simulink model "Simulink_System2"  (R2020a)
settings: Solver=VariableStepAuto  StartTime=0.0  StopTime=50  MaxStep=0.001  RelTol=1e-3
undefined symbols (not defined in the file): a, k2, kcA2, kcSO2, kdA2, kdSO2, kiA2, kiSO2
libraries: cstblocks x4, simulink x1
settings Model: Creator=beto1  LastModifiedBy=beto1

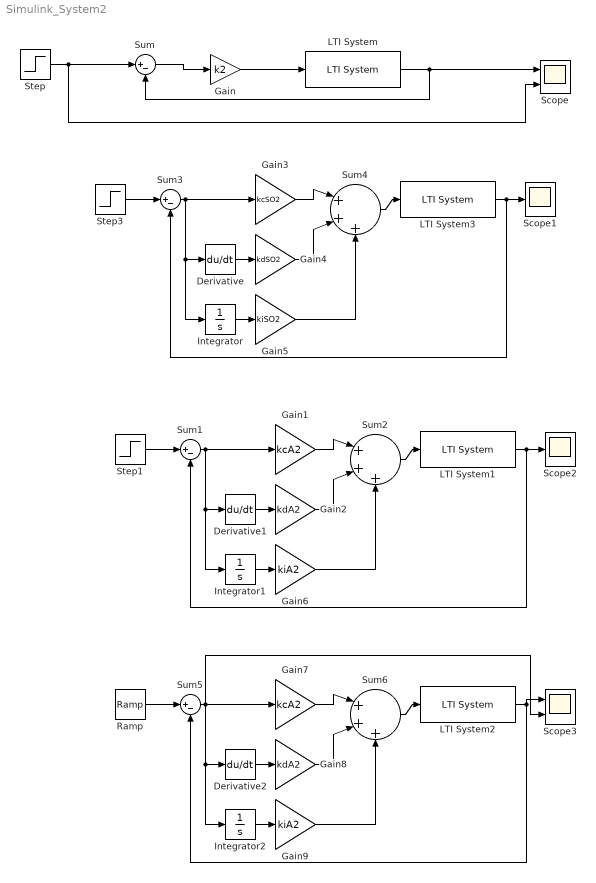
== system Simulink_System2 ==
  Derivative : Derivative
  Derivative1 : Derivative
  Derivative2 : Derivative
  Gain : Gain  Gain=k2
  Gain1 : Gain  Gain=kcA2
  Gain2 : Gain  Gain=kdA2
  Gain3 : Gain  Gain=kcSO2
  Gain4 : Gain  Gain=kdSO2
  Gain5 : Gain  Gain=kiSO2
  Gain6 : Gain  Gain=kiA2
  Gain7 : Gain  Gain=kcA2
  Gain8 : Gain  Gain=kdA2
  Gain9 : Gain  Gain=kiA2
  Integrator : Integrator
  Integrator1 : Integrator
  Integrator2 : Integrator
  LTI System{,1..3} (4 alike) : cstblocks/LTI System  sys=G2  IC=[]
  Ramp : simulink/Sources/Ramp  slope=a  start=0  InitialOutput=0
  Scope : Scope  NumInputPorts=2
  Scope1 : Scope
  Scope2 : Scope
  Scope3 : Scope  NumInputPorts=2
  Step : Step  Time=0  SampleTime=0
  Step1 : Step  Time=0  After=8  SampleTime=0
  Step3 : Step  Time=0  After=8  SampleTime=0
  Sum{,1,3,5} (4 alike) : Sum  Inputs=|+-
  Sum2 : Sum  Inputs=|+++
  Sum4 : Sum  Inputs=|+++
  Sum6 : Sum  Inputs=|+++
  wires:
  LTI System/1 -> Sum/2, Scope/1
  Sum/1 -> Gain/1
  Gain/1 -> LTI System/1
  Step/1 -> Sum/1, Scope/2
  Gain5/1 -> Sum4/3
  Derivative/1 -> Gain4/1
  Integrator/1 -> Gain5/1
  Sum3/1 -> Integrator/1, Derivative/1, Gain3/1
  Gain3/1 -> Sum4/1
  LTI System3/1 -> Sum3/2, Scope1/1
  Sum4/1 -> LTI System3/1
  Step3/1 -> Sum3/1
  Gain4/1 -> Sum4/2
  Gain6/1 -> Sum2/3
  Derivative1/1 -> Gain2/1
  Integrator1/1 -> Gain6/1
  Sum1/1 -> Integrator1/1, Derivative1/1, Gain1/1
  Gain1/1 -> Sum2/1
  LTI System1/1 -> Sum1/2, Scope2/1
  Sum2/1 -> LTI System1/1
  Step1/1 -> Sum1/1
  Gain2/1 -> Sum2/2
  Integrator2/1 -> Gain9/1
  Gain9/1 -> Sum6/3
  Derivative2/1 -> Gain8/1
  Gain8/1 -> Sum6/2
  Sum6/1 -> LTI System2/1
  Gain7/1 -> Sum6/1
  LTI System2/1 -> Sum5/2, Scope3/1
  Ramp/1 -> Sum5/1
  Sum5/1 -> Scope3/2, Integrator2/1, Derivative2/1, Gain7/1
